simulink model "Dynamics"  (R2018a)
settings: Solver=FixedStepDiscrete  StartTime=0.0  StopTime=10.0  FixedStep=.01  RelTol=1e-3
undefined symbols (not defined in the file): Ts
libraries: aerolibutil x5, vrlib x4
settings Model: Creator=henry  LastModifiedBy=henry

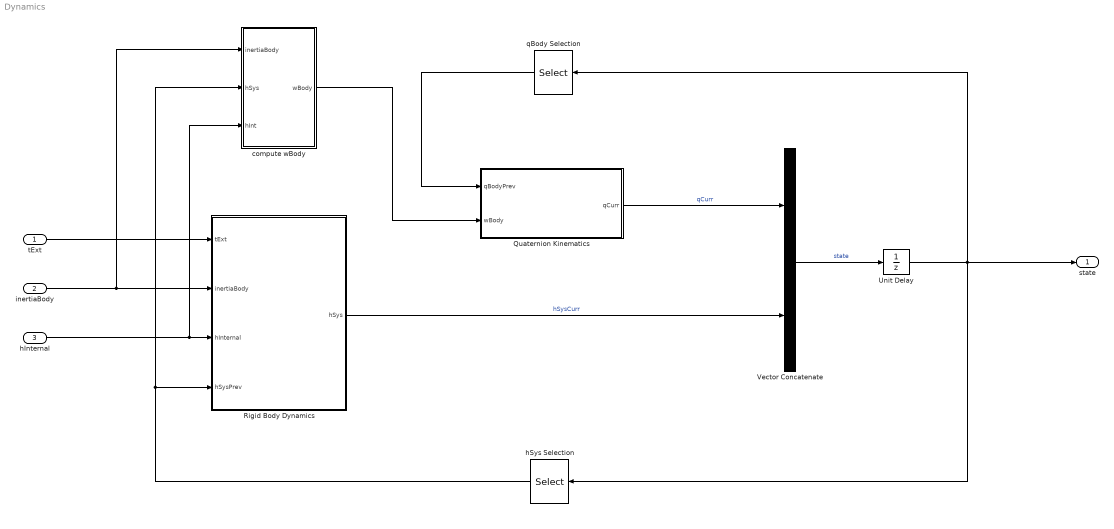
== system Dynamics ==
  tExt : Inport
  inertiaBody : Inport  Port=2
  hInternal : Inport  Port=3
  Quaternion Kinematics : Subsystem
  Rigid Body Dynamics : Subsystem
  Unit Delay : UnitDelay  SampleTime=-1
  Vector Concatenate : Concatenate
  compute wBody : Subsystem
  hSys Selection : Selector  InputPortWidth=6  IndexOptions=Index vector (dialog)  Indices=[4:6]  OutputSizes=1
  qBody Selection : Selector  InputPortWidth=6  IndexOptions=Index vector (dialog)  Indices=[1:3]  OutputSizes=1
  state : Outport
  wires:
  Unit Delay/1 -> state/1, hSys Selection/1, qBody Selection/1
  Vector Concatenate/1 -> Unit Delay/1  "state"
  Quaternion Kinematics/1(qCurr) -> Vector Concatenate/1  "qCurr"
  Rigid Body Dynamics/1(hSys) -> Vector Concatenate/2  "hSysCurr"
  qBody Selection/1 -> Quaternion Kinematics/1(qBodyPrev)
  hSys Selection/1 -> compute wBody/2(hSys), Rigid Body Dynamics/4(hSysPrev)
  tExt/1 -> Rigid Body Dynamics/1(tExt)
  inertiaBody/1 -> compute wBody/1(inertiaBody), Rigid Body Dynamics/2(inertiaBody)
  hInternal/1 -> compute wBody/3(hInt), Rigid Body Dynamics/3(hInternal)
  compute wBody/1(wBody) -> Quaternion Kinematics/2(wBody)

== system Dynamics/Quaternion Kinematics ==
  qBodyPrev : Inport
  wBody : Inport  Port=2
  Terminator : Terminator
  qCurr : Outport
  wires:
  wBody/1 -> Terminator/1
  qBodyPrev/1 -> qCurr/1

== system Dynamics/Rigid Body Dynamics ==
  tExt : Inport
  inertiaBody : Inport  Port=2
  hInternal : Inport  Port=3
  hSysPrev : Inport  Port=4
  rk45 integrator : Subsystem
  hSys : Outport
  wires:
  tExt/1 -> rk45 integrator/1(tExt)
  inertiaBody/1 -> rk45 integrator/2(inertiaBody)
  hSysPrev/1 -> rk45 integrator/3(hSysInit)
  hInternal/1 -> rk45 integrator/4(hInternal)
  rk45 integrator/1(hSys) -> hSys/1

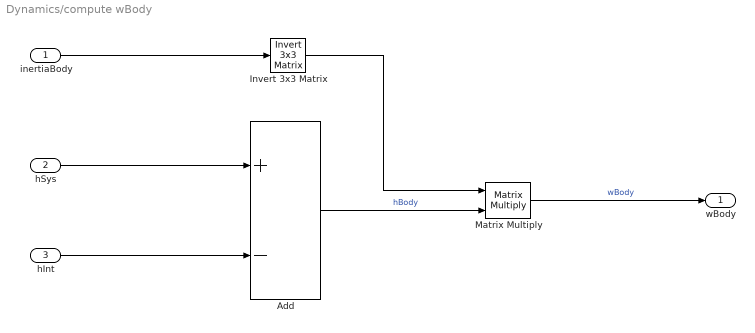
== system Dynamics/compute wBody ==
  inertiaBody : Inport
  hSys : Inport  Port=2
  hInt : Inport  Port=3
  Add : Sum  Inputs=+-
  Invert 3x3 Matrix : aerolibutil/Invert  3x3 Matrix
  Matrix Multiply : Product  Multiplication=Matrix(*)
  wBody : Outport
  wires:
  inertiaBody/1 -> Invert 3x3 Matrix/1
  hSys/1 -> Add/1
  Matrix Multiply/1 -> wBody/1  "wBody"
  Invert 3x3 Matrix/1 -> Matrix Multiply/1
  hInt/1 -> Add/2
  Add/1 -> Matrix Multiply/2  "hBody"

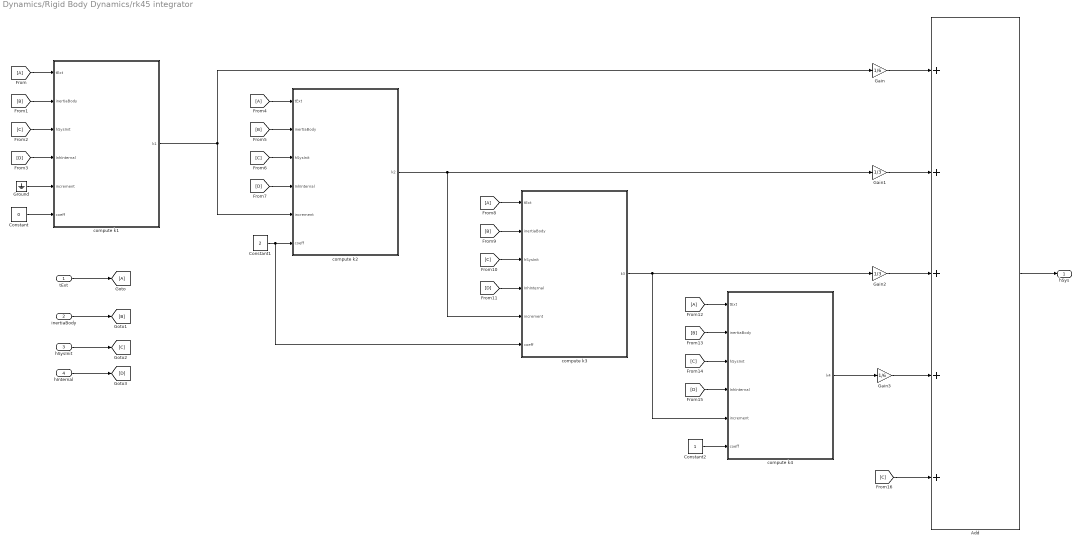
== system Dynamics/Rigid Body Dynamics/rk45 integrator ==
  tExt : Inport
  inertiaBody : Inport  Port=2
  hSysInit : Inport  Port=3
  hInternal : Inport  Port=4
  Add : Sum  Inputs=+++++
  Constant : Constant  Value=0
  Constant1 : Constant  Value=2
  Constant2 : Constant
  Gain : Gain  Gain=1/6
  Gain1 : Gain  Gain=1/3
  Gain2 : Gain  Gain=1/3
  Gain3 : Gain  Gain=1/6
  Ground : Ground
  compute k1 : Subsystem
  compute k2 : Subsystem
  compute k3 : Subsystem
  compute k4 : Subsystem
  hSys : Outport
  wires:
  Ground/1 -> compute k1/5(increment)
  Constant/1 -> compute k1/6(coeff)
  [A] -> compute k1/1(tExt)
  tExt/1 -> [A]
  inertiaBody/1 -> [B]
  hSysInit/1 -> [C]
  hInternal/1 -> [D]
  [B] -> compute k1/2(inertiaBody)
  [C] -> compute k1/3(hSysInit)
  [D] -> compute k1/4(InhInternal)
  [B] -> compute k2/2(inertiaBody)
  [D] -> compute k2/4(InhInternal)
  [A] -> compute k2/1(tExt)
  [C] -> compute k2/3(hSysInit)
  [B] -> compute k3/2(inertiaBody)
  [D] -> compute k3/4(InhInternal)
  [A] -> compute k3/1(tExt)
  [C] -> compute k3/3(hSysInit)
  [B] -> compute k4/2(inertiaBody)
  [D] -> compute k4/4(InhInternal)
  [A] -> compute k4/1(tExt)
  [C] -> compute k4/3(hSysInit)
  compute k1/1(k1) -> compute k2/5(increment), Gain/1
  compute k2/1(k2) -> compute k3/5(increment), Gain1/1
  compute k3/1(k3) -> compute k4/5(increment), Gain2/1
  Constant2/1 -> compute k4/6(coeff)
  Constant1/1 -> compute k3/6(coeff), compute k2/6(coeff)
  compute k4/1(k4) -> Gain3/1
  Gain/1 -> Add/1
  Gain1/1 -> Add/2
  Gain2/1 -> Add/3
  Gain3/1 -> Add/4
  [C] -> Add/5
  Add/1 -> hSys/1

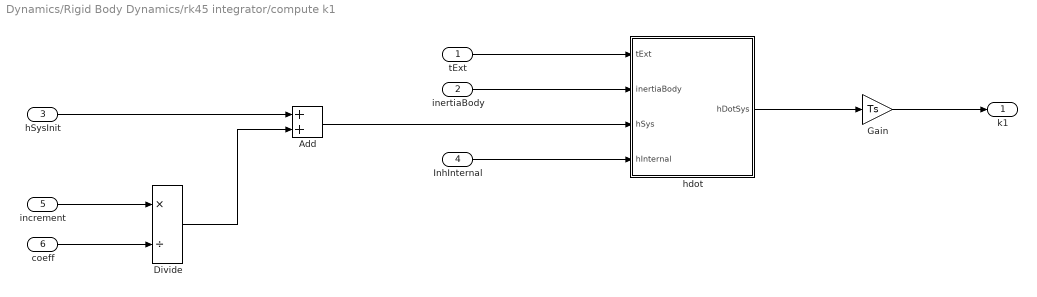
== system Dynamics/Rigid Body Dynamics/rk45 integrator/compute k1 ==
  tExt : Inport
  inertiaBody : Inport  Port=2
  hSysInit : Inport  Port=3
  InhInternal : Inport  Port=4
  increment : Inport  Port=5
  coeff : Inport  Port=6
  Add : Sum
  Divide : Product  Inputs=*/
  Gain : Gain  Gain=Ts
  hdot : Subsystem
  k1 : Outport
  wires:
  InhInternal/1 -> hdot/4(hInternal)
  inertiaBody/1 -> hdot/2(inertiaBody)
  tExt/1 -> hdot/1(tExt)
  hSysInit/1 -> Add/1
  increment/1 -> Divide/1
  coeff/1 -> Divide/2
  Divide/1 -> Add/2
  Add/1 -> hdot/3(hSys)
  hdot/1(hDotSys) -> Gain/1
  Gain/1 -> k1/1

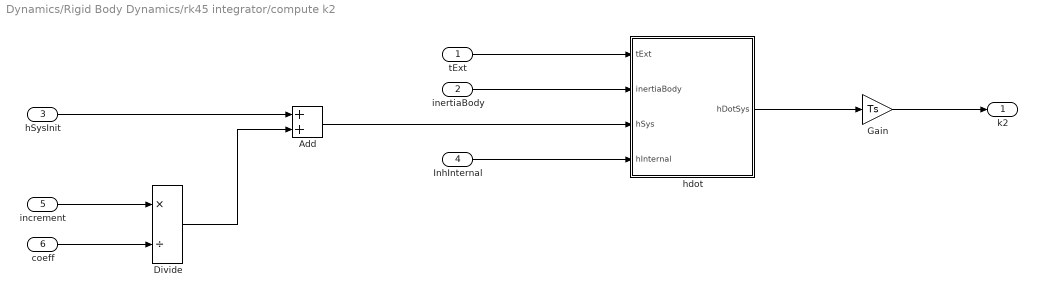
== system Dynamics/Rigid Body Dynamics/rk45 integrator/compute k2 ==
  tExt : Inport
  inertiaBody : Inport  Port=2
  hSysInit : Inport  Port=3
  InhInternal : Inport  Port=4
  increment : Inport  Port=5
  coeff : Inport  Port=6
  Add : Sum
  Divide : Product  Inputs=*/
  Gain : Gain  Gain=Ts
  hdot : Subsystem
  k2 : Outport
  wires:
  InhInternal/1 -> hdot/4(hInternal)
  inertiaBody/1 -> hdot/2(inertiaBody)
  tExt/1 -> hdot/1(tExt)
  hSysInit/1 -> Add/1
  increment/1 -> Divide/1
  coeff/1 -> Divide/2
  Divide/1 -> Add/2
  Add/1 -> hdot/3(hSys)
  hdot/1(hDotSys) -> Gain/1
  Gain/1 -> k2/1

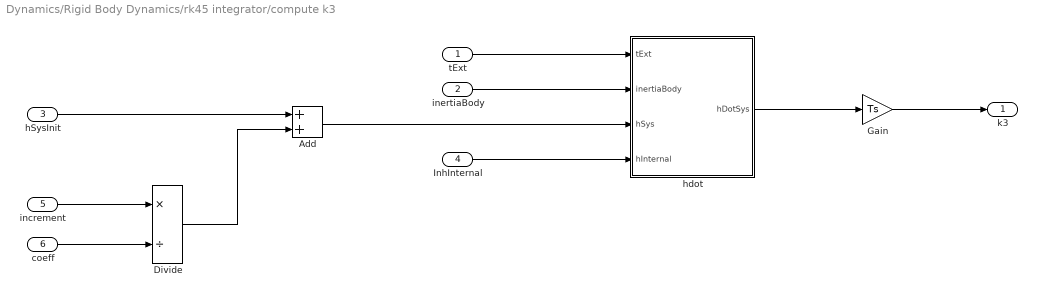
== system Dynamics/Rigid Body Dynamics/rk45 integrator/compute k3 ==
  tExt : Inport
  inertiaBody : Inport  Port=2
  hSysInit : Inport  Port=3
  InhInternal : Inport  Port=4
  increment : Inport  Port=5
  coeff : Inport  Port=6
  Add : Sum
  Divide : Product  Inputs=*/
  Gain : Gain  Gain=Ts
  hdot : Subsystem
  k3 : Outport
  wires:
  InhInternal/1 -> hdot/4(hInternal)
  inertiaBody/1 -> hdot/2(inertiaBody)
  tExt/1 -> hdot/1(tExt)
  hSysInit/1 -> Add/1
  increment/1 -> Divide/1
  coeff/1 -> Divide/2
  Divide/1 -> Add/2
  Add/1 -> hdot/3(hSys)
  hdot/1(hDotSys) -> Gain/1
  Gain/1 -> k3/1

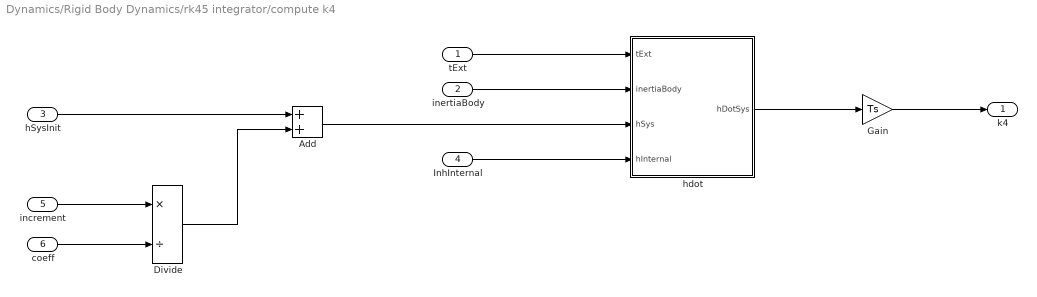
== system Dynamics/Rigid Body Dynamics/rk45 integrator/compute k4 ==
  tExt : Inport
  inertiaBody : Inport  Port=2
  hSysInit : Inport  Port=3
  InhInternal : Inport  Port=4
  increment : Inport  Port=5
  coeff : Inport  Port=6
  Add : Sum
  Divide : Product  Inputs=*/
  Gain : Gain  Gain=Ts
  hdot : Subsystem
  k4 : Outport
  wires:
  InhInternal/1 -> hdot/4(hInternal)
  inertiaBody/1 -> hdot/2(inertiaBody)
  tExt/1 -> hdot/1(tExt)
  hSysInit/1 -> Add/1
  increment/1 -> Divide/1
  coeff/1 -> Divide/2
  Divide/1 -> Add/2
  Add/1 -> hdot/3(hSys)
  hdot/1(hDotSys) -> Gain/1
  Gain/1 -> k4/1

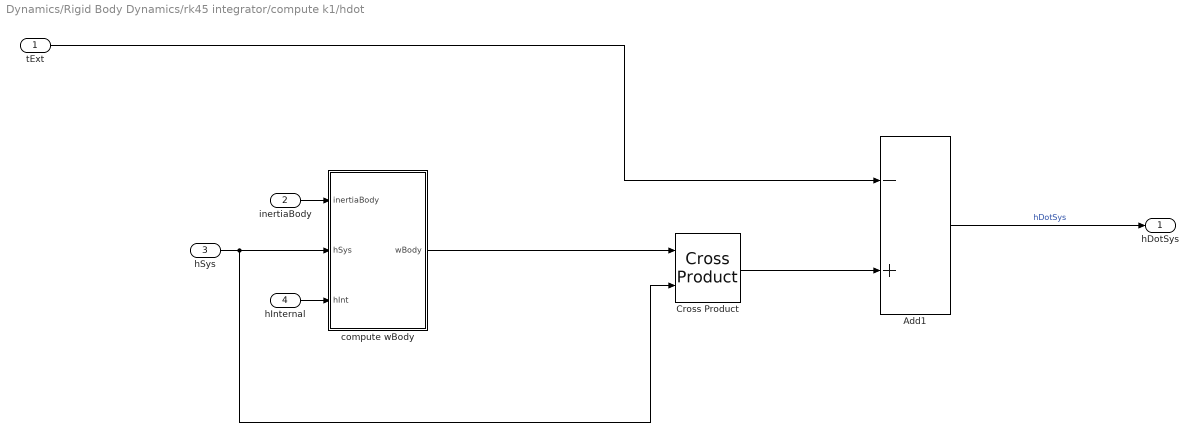
== system Dynamics/Rigid Body Dynamics/rk45 integrator/compute k1/hdot ==
  tExt : Inport
  inertiaBody : Inport  Port=2
  hSys : Inport  Port=3
  hInternal : Inport  Port=4
  Add1 : Sum  Inputs=-+
  Cross Product : vrlib/Utilities/Cross Product
      settings: SourceProductBaseCode=VR
  compute wBody : Subsystem
  hDotSys : Outport
  wires:
  Add1/1 -> hDotSys/1  "hDotSys"
  tExt/1 -> Add1/1
  Cross Product/1 -> Add1/2
  inertiaBody/1 -> compute wBody/1(inertiaBody)
  hInternal/1 -> compute wBody/3(hInt)
  compute wBody/1(wBody) -> Cross Product/1
  hSys/1 -> Cross Product/2, compute wBody/2(hSys)

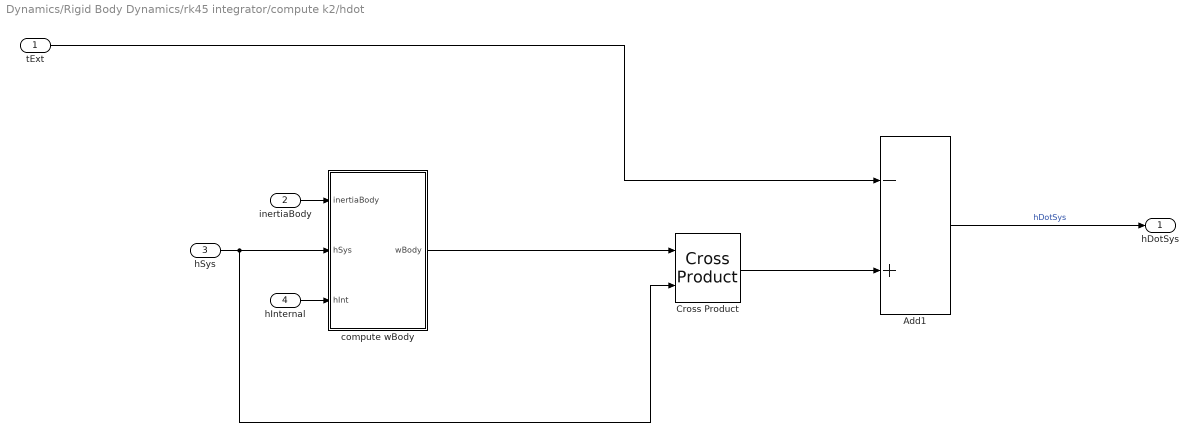
== system Dynamics/Rigid Body Dynamics/rk45 integrator/compute k2/hdot ==
  tExt : Inport
  inertiaBody : Inport  Port=2
  hSys : Inport  Port=3
  hInternal : Inport  Port=4
  Add1 : Sum  Inputs=-+
  Cross Product : vrlib/Utilities/Cross Product
      settings: SourceProductBaseCode=VR
  compute wBody : Subsystem
  hDotSys : Outport
  wires:
  Add1/1 -> hDotSys/1  "hDotSys"
  tExt/1 -> Add1/1
  Cross Product/1 -> Add1/2
  inertiaBody/1 -> compute wBody/1(inertiaBody)
  hInternal/1 -> compute wBody/3(hInt)
  compute wBody/1(wBody) -> Cross Product/1
  hSys/1 -> Cross Product/2, compute wBody/2(hSys)

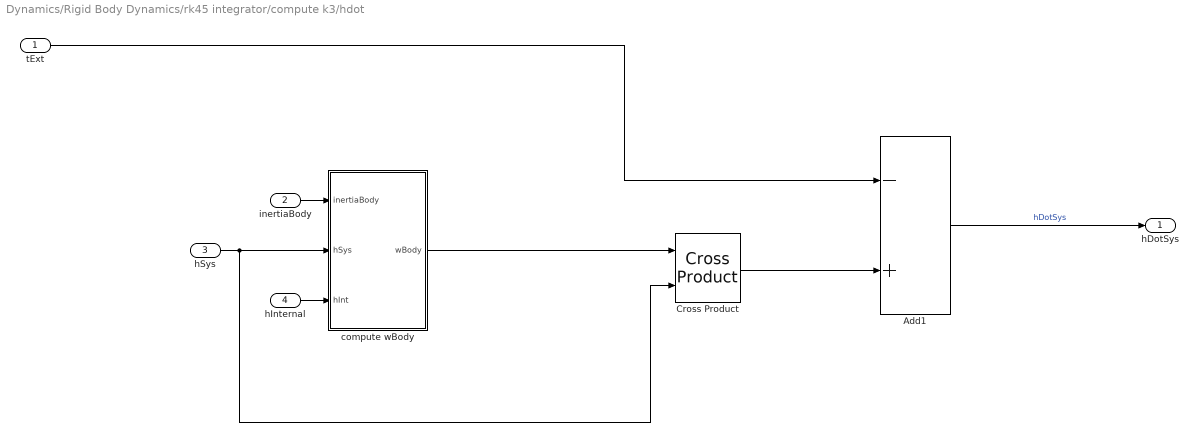
== system Dynamics/Rigid Body Dynamics/rk45 integrator/compute k3/hdot ==
  tExt : Inport
  inertiaBody : Inport  Port=2
  hSys : Inport  Port=3
  hInternal : Inport  Port=4
  Add1 : Sum  Inputs=-+
  Cross Product : vrlib/Utilities/Cross Product
      settings: SourceProductBaseCode=VR
  compute wBody : Subsystem
  hDotSys : Outport
  wires:
  Add1/1 -> hDotSys/1  "hDotSys"
  tExt/1 -> Add1/1
  Cross Product/1 -> Add1/2
  inertiaBody/1 -> compute wBody/1(inertiaBody)
  hInternal/1 -> compute wBody/3(hInt)
  compute wBody/1(wBody) -> Cross Product/1
  hSys/1 -> Cross Product/2, compute wBody/2(hSys)

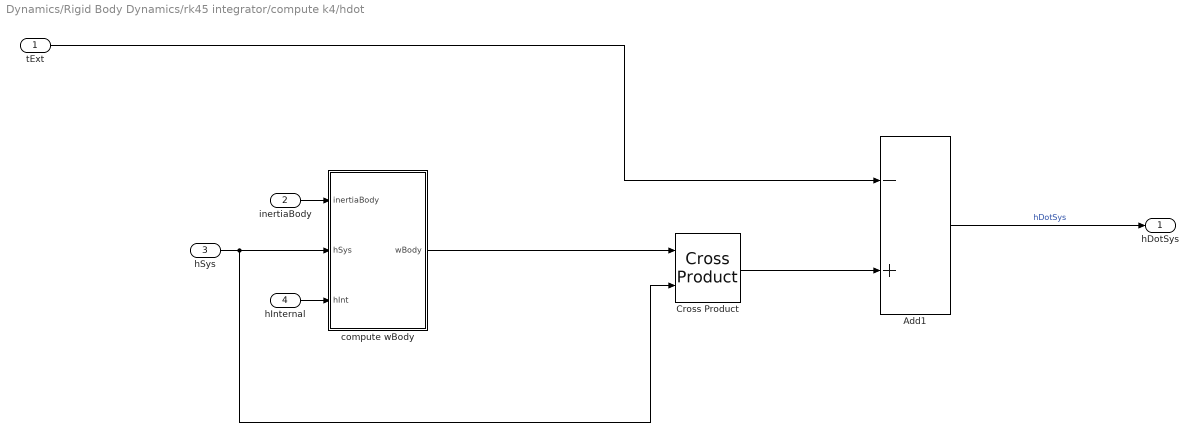
== system Dynamics/Rigid Body Dynamics/rk45 integrator/compute k4/hdot ==
  tExt : Inport
  inertiaBody : Inport  Port=2
  hSys : Inport  Port=3
  hInternal : Inport  Port=4
  Add1 : Sum  Inputs=-+
  Cross Product : vrlib/Utilities/Cross Product
      settings: SourceProductBaseCode=VR
  compute wBody : Subsystem
  hDotSys : Outport
  wires:
  Add1/1 -> hDotSys/1  "hDotSys"
  tExt/1 -> Add1/1
  Cross Product/1 -> Add1/2
  inertiaBody/1 -> compute wBody/1(inertiaBody)
  hInternal/1 -> compute wBody/3(hInt)
  compute wBody/1(wBody) -> Cross Product/1
  hSys/1 -> Cross Product/2, compute wBody/2(hSys)

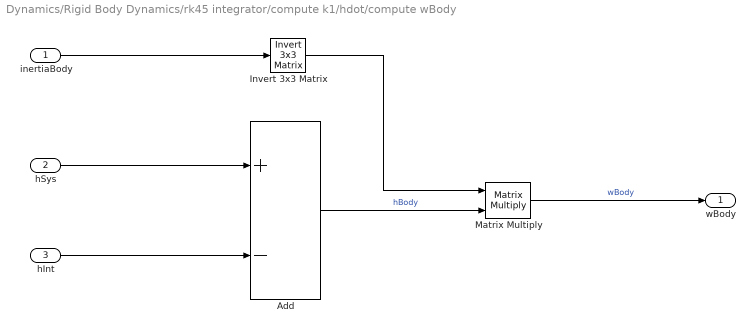
== system Dynamics/Rigid Body Dynamics/rk45 integrator/compute k1/hdot/compute wBody ==
  inertiaBody : Inport
  hSys : Inport  Port=2
  hInt : Inport  Port=3
  Add : Sum  Inputs=+-
  Invert 3x3 Matrix : aerolibutil/Invert  3x3 Matrix
  Matrix Multiply : Product  Multiplication=Matrix(*)
  wBody : Outport
  wires:
  inertiaBody/1 -> Invert 3x3 Matrix/1
  hSys/1 -> Add/1
  Matrix Multiply/1 -> wBody/1  "wBody"
  Invert 3x3 Matrix/1 -> Matrix Multiply/1
  hInt/1 -> Add/2
  Add/1 -> Matrix Multiply/2  "hBody"

== system Dynamics/Rigid Body Dynamics/rk45 integrator/compute k2/hdot/compute wBody ==
  inertiaBody : Inport
  hSys : Inport  Port=2
  hInt : Inport  Port=3
  Add : Sum  Inputs=+-
  Invert 3x3 Matrix : aerolibutil/Invert  3x3 Matrix
  Matrix Multiply : Product  Multiplication=Matrix(*)
  wBody : Outport
  wires:
  inertiaBody/1 -> Invert 3x3 Matrix/1
  hSys/1 -> Add/1
  Matrix Multiply/1 -> wBody/1  "wBody"
  Invert 3x3 Matrix/1 -> Matrix Multiply/1
  hInt/1 -> Add/2
  Add/1 -> Matrix Multiply/2  "hBody"

== system Dynamics/Rigid Body Dynamics/rk45 integrator/compute k3/hdot/compute wBody ==
  inertiaBody : Inport
  hSys : Inport  Port=2
  hInt : Inport  Port=3
  Add : Sum  Inputs=+-
  Invert 3x3 Matrix : aerolibutil/Invert  3x3 Matrix
  Matrix Multiply : Product  Multiplication=Matrix(*)
  wBody : Outport
  wires:
  inertiaBody/1 -> Invert 3x3 Matrix/1
  hSys/1 -> Add/1
  Matrix Multiply/1 -> wBody/1  "wBody"
  Invert 3x3 Matrix/1 -> Matrix Multiply/1
  hInt/1 -> Add/2
  Add/1 -> Matrix Multiply/2  "hBody"

== system Dynamics/Rigid Body Dynamics/rk45 integrator/compute k4/hdot/compute wBody ==
  inertiaBody : Inport
  hSys : Inport  Port=2
  hInt : Inport  Port=3
  Add : Sum  Inputs=+-
  Invert 3x3 Matrix : aerolibutil/Invert  3x3 Matrix
  Matrix Multiply : Product  Multiplication=Matrix(*)
  wBody : Outport
  wires:
  inertiaBody/1 -> Invert 3x3 Matrix/1
  hSys/1 -> Add/1
  Matrix Multiply/1 -> wBody/1  "wBody"
  Invert 3x3 Matrix/1 -> Matrix Multiply/1
  hInt/1 -> Add/2
  Add/1 -> Matrix Multiply/2  "hBody"
